simulink model "rigid_launcher_syn"  (R2025a)
settings: Solver=VariableStepAuto  StartTime=0.0  StopTime=10.0  RelTol=1e-3
undefined symbols (not defined in the file or in its folder): Ar, Br, Cr, Dr
settings Model: Creator=asus  LastModifiedBy=asus
settings OptimizationCC: DefaultParameterBehavior=Inlined
settings DebuggingCC: InitInArrayFormatMsg=none

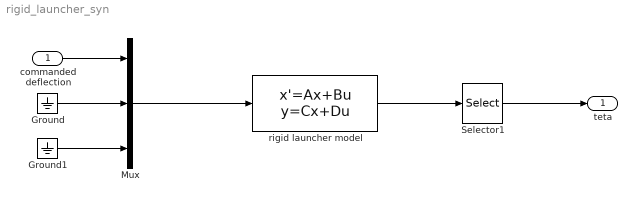
== system rigid_launcher_syn ==
  commanded deflection : Inport
  Ground : Ground
  Ground1 : Ground
  Mux : Mux  Inputs=3
  Selector1 : Selector  InputPortWidth=6  IndexOptions=Index vector (dialog)  Indices=[2]  OutputSizes=1
  rigid launcher model : StateSpace  A=Ar  B=Br  C=Cr  D=Dr  InitialCondition=0
  teta : Outport
  wires:
  commanded deflection/1 -> Mux/1
  Mux/1 -> rigid launcher model/1
  rigid launcher model/1 -> Selector1/1
  Ground/1 -> Mux/2
  Ground1/1 -> Mux/3
  Selector1/1 -> teta/1
